simulink model "Events"  (Simulink 7.4)
settings: Solver=ode45  StartTime=0.0  StopTime=10.0  RelTol=1e-3
settings Model: Creator=dread  LastModifiedBy=dread

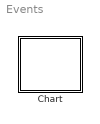
== system Events ==
  Chart : Stateflow chart

== stateflow chart Chart ==
  state State
    state SubState
      state SubSubState
  events: stateEvent local EITHER_EDGE_EVENT; subStateEvent local EITHER_EDGE_EVENT; subSubStateEvent local EITHER_EDGE_EVENT; chartEvent local EITHER_EDGE_EVENT
